simulink model "punto_4"  (Simulink 7.5)
settings: Solver=ode45  StartTime=0.0  StopTime=3  RelTol=1e-3
settings Model: Creator=davito  LastModifiedBy=davito

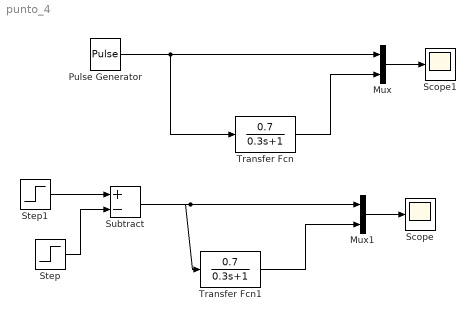
== system punto_4 ==
  Mux : Mux  Inputs=2
  Mux1 : Mux  Inputs=2
  Pulse Generator : DiscretePulseGenerator  PulseType=Time based  Amplitude=10  Period=10  PulseWidth=10  PhaseDelay=0  SampleTime=1
  Scope : Scope
      settings: TimeRange=3  YMin=-0.5  YMax=10.5
  Scope1 : Scope
      settings: TimeRange=5  YMin=0  YMax=10
  Step : Step  After=10  SampleTime=0
  Step1 : Step  Time=0  After=10  SampleTime=0
  Subtract : Sum  Inputs=+-  OutDataType=fixdt(1, 16)  OutScaling=2^-10
  Transfer Fcn : TransferFcn  Numerator=[0.7]  Denominator=[0.3 1]
  Transfer Fcn1 : TransferFcn  Numerator=[0.7]  Denominator=[0.3 1]
  wires:
  Pulse Generator/1 -> Mux/1, Transfer Fcn/1
  Transfer Fcn/1 -> Mux/2
  Mux/1 -> Scope1/1
  Step/1 -> Subtract/2
  Step1/1 -> Subtract/1
  Mux1/1 -> Scope/1
  Subtract/1 -> Mux1/1, Transfer Fcn1/1
  Transfer Fcn1/1 -> Mux1/2
